simulink model "LEO_EMC_System"  (R2021a)
settings: Solver=FixedStepDiscrete  StartTime=0.0  StopTime=10  FixedStep=1000/15.36e6  RelTol=1e-3
undefined symbols (not defined in the file or in its folder): bp_time, table_dop, table_pl
settings Model: Creator=52834  LastModifiedBy=52834

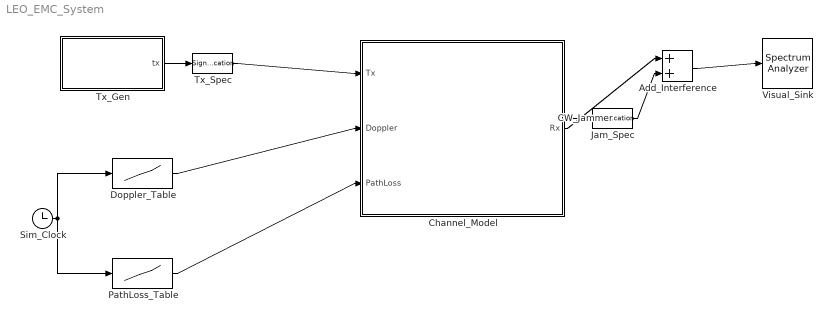
== system LEO_EMC_System ==
  Add_Interference : Sum
  CW_Jammer : MATLAB Function  TreatAsAtomicUnit=on
  Channel_Model : Subsystem
  Doppler_Table : Lookup_n-D  NumberOfTableDimensions=1  BreakpointsForDimension1=bp_time  Table=table_dop  ExtrapMethod=Clip  InternalRulePriority=Speed  RndMeth=Simplest  InputSameDT=on
  Jam_Spec : SignalSpecification  Dimensions=[1000 1]
      settings: SignalType=complex
  PathLoss_Table : Lookup_n-D  NumberOfTableDimensions=1  BreakpointsForDimension1=bp_time  Table=table_pl  ExtrapMethod=Clip  InternalRulePriority=Speed  RndMeth=Simplest  InputSameDT=on
  Sim_Clock : Clock
  Tx_Gen : MATLAB Function  TreatAsAtomicUnit=on
  Tx_Spec : SignalSpecification  Dimensions=[1000 1]
      settings: SignalType=complex
  Visual_Sink : SpectrumAnalyzer  IOType=viewer
  wires:
  Tx_Gen/1(tx) -> Tx_Spec/1
  Tx_Spec/1 -> Channel_Model/1(Tx)
  Sim_Clock/1 -> Doppler_Table/1, PathLoss_Table/1
  Doppler_Table/1 -> Channel_Model/2(Doppler)
  PathLoss_Table/1 -> Channel_Model/3(PathLoss)
  Channel_Model/1(Rx) -> Add_Interference/1
  CW_Jammer/1(y) -> Jam_Spec/1
  Jam_Spec/1 -> Add_Interference/2
  Add_Interference/1 -> Visual_Sink/1

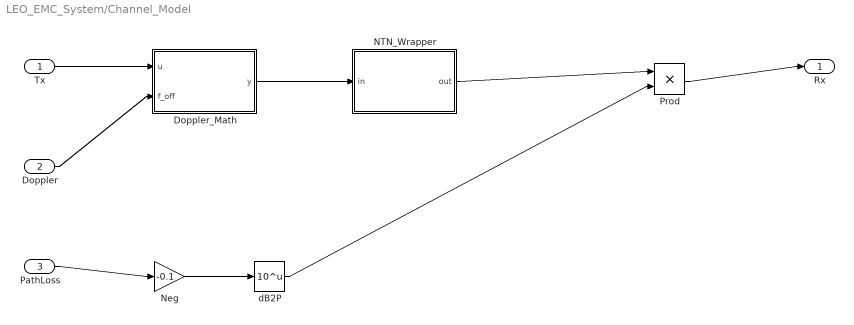
== system LEO_EMC_System/Channel_Model ==
  Tx : Inport
  Doppler : Inport  Port=2
  PathLoss : Inport  Port=3
  Doppler_Math : MATLAB Function  TreatAsAtomicUnit=on
  NTN_Wrapper : MATLAB Function  TreatAsAtomicUnit=on
  Neg : Gain  Gain=-0.1
  Prod : Product
  dB2P : Math  Operator=10^u  SaturateOnIntegerOverflow=on
  Rx : Outport
  wires:
  Tx/1 -> Doppler_Math/1(u)
  Doppler/1 -> Doppler_Math/2(f_off)
  Doppler_Math/1(y) -> NTN_Wrapper/1(in)
  PathLoss/1 -> Neg/1
  Neg/1 -> dB2P/1
  NTN_Wrapper/1(out) -> Prod/1
  dB2P/1 -> Prod/2
  Prod/1 -> Rx/1

== matlab function LEO_EMC_System/Tx_Gen ==
  data: tx output
function tx = fcn()
 persistent wave idx
 FRAME_SIZE=1000;
coder.varsize('tx', [1000 1], [0 0]);
if isempty(wave), rng(1); d=complex(randn(3e5,1),randn(3e5,1)); wave=d/max(abs(d)); idx=1; end
if idx+FRAME_SIZE-1>length(wave), idx=1; end
tx=complex(zeros(FRAME_SIZE,1)); tx(:)=wave(idx:idx+FRAME_SIZE-1); idx=idx+FRAME_SIZE;

== matlab function LEO_EMC_System/Channel_Model/NTN_Wrapper ==
  data: in input; out output
function out = fcn(in)
 persistent h
 coder.varsize('out',[1000 1],[0 0]);
if isempty(h), h=nrTDLChannel(); h.DelayProfile='Custom'; h.PathDelays=[0 1e-7 2e-7];
h.AveragePathGains=[0 -4 -6]; h.NumTransmitAntennas=1; h.NumReceiveAntennas=1; h.SampleRate=15.36e6; end
[out,~]=h(in);

== matlab function LEO_EMC_System/CW_Jammer ==
  data: y output
function y = fcn()
 persistent p
 coder.varsize('y',[1000 1],[0 0]);
if isempty(p), p=0; end
 Fs=15.36e6; t=(0:999).'/Fs; y=complex(zeros(1000,1));
y(:)=0.1*exp(1i*(p+2*pi*100*t)); p=mod(p+2*pi*100*(1000/Fs),2*pi);

== matlab function LEO_EMC_System/Channel_Model/Doppler_Math ==
  data: u input; y output; f_off input
function y = fcn(u, f_off)
 persistent lp
 coder.varsize('y',[1000 1],[0 0]);
if isempty(lp), lp=0; end
 Ts=1/15.36e6; t=(1:1000).'*Ts;
inc=2*pi*f_off*t; y=u.*exp(1i*(lp+inc)); lp=mod(lp+inc(end),2*pi);
